simulink model "ActuatorLoop"  (R2019b)
settings: Solver=FixedStepDiscrete  StartTime=0.0  StopTime=10.0  FixedStep=0.001  RelTol=1e-3  EnableMultiTasking=on
model workspace (MAT data in the model file):
  Kd = Simulink.Parameter
  Kd.Value = 0.00272
  Kd.DataType = 'double'
  Kd.Dimensions = [1 1]
  Ki = Simulink.Parameter
  Ki.Value = 2.73
  Ki.DataType = 'double'
  Ki.Dimensions = [1 1]
  Kp = Simulink.Parameter
  Kp.Value = 0.339
  Kp.DataType = 'double'
  Kp.Dimensions = [1 1]
undefined symbols (not defined in the file or in its folder): DiscIntNeverNeededParam
libraries: simulink x2
Description:
  | This model implements a proportional, integral, derivative controller to close the loop on a hydraulic actuator.
settings Model: RequirementInfo="{}  %GIDa_c39459e1_b1c4_416b_a121_7cdfa8af617e"  DataDictionary=HeliSystemDD.sldd  ParameterArgumentNames=Kp,Kd,Ki  Creator=bpotter  LastModifiedBy=bpotter
settings DataIOCC: LimitDataPoints=on  SaveFormat=Array  SaveOutput=off  SignalLogging=off  DSMLogging=off  SaveTime=off
settings OptimizationCC: BlockReduction=off  DefaultParameterBehavior=Inlined  UseDivisionForNetSlopeComputation=on  InlineInvariantSignals=on  InitFltsAndDblsToZero=on  EfficientFloat2IntCast=on  EfficientMapNaN2IntZero=off  LifeSpan=inf  MaxStackSize=inf  EfficientTunableParamExpr=on
settings DebuggingCC: SignalInfNanChecking=error  SignalRangeChecking=error  ReadBeforeWriteMsg=EnableAllAsError  WriteAfterWriteMsg=EnableAllAsError  WriteAfterReadMsg=EnableAllAsError  AlgebraicLoopMsg=error  ArtificialAlgebraicLoopMsg=error  SaveWithDisabledLinksMsg=error  SaveWithParameterizedLinksMsg=error  BlockPriorityViolationMsg=error  SolverPrmCheckMsg=error  InheritedTsInSrcMsg=error  SingleTaskRateTransMsg=error  TasksWithSamePriorityMsg=error  SigSpecEnsureSampleTimeMsg=error  CheckMatrixSingularityMsg=error  IntegerOverflowMsg=error  ParameterUnderflowMsg=error  ParameterPrecisionLossMsg=error  ParameterTunabilityLossMsg=error  UnderSpecifiedDataTypeMsg=error  UnnecessaryDatatypeConvMsg=warning  VectorMatrixConversionMsg=error  SignalLabelMismatchMsg=error  UnconnectedInputMsg=error  UnconnectedOutputMsg=error  UnconnectedLineMsg=error  SFcnCompatibilityMsg=error  UniqueDataStoreMsg=error  BusObjectLabelMismatch=error  RootOutportRequireBusObject=error  AssertControl=DisableAll  AllowSymbolicDim=off  ModelReferenceIOMsg=error  ModelReferenceIOMismatchMessage=error  UnknownTsInhSupMsg=error  ModelReferenceDataLoggingMessage=error  StateNameClashWarn=warning  PregeneratedLibrarySubsystemCodeDiagnostic=none  StrictBusMsg=ErrorOnBusTreatedAsVector  NonBusSignalsTreatedAsBus=error  SFInvalidInputDataAccessInChartInitDiag=error  SFTransitionOutsideNaturalParentDiag=error  SFUnreachableExecutionPathDiag=error  SFUndirectedBroadcastEventsDiag=error  SFTransitionActionBeforeConditionDiag=error  SFExecutionAtInitializationDiag=none  IntegerSaturationMsg=error  ArithmeticOperatorsInVariantConditions=warning
settings HardwareCC: ProdBitPerPointer=32  ProdBitPerSizeT=32  ProdBitPerPtrDiffT=32  ProdWordSize=32  ProdHWDeviceType=Intel->x86-32 (Windows32)
settings ModelReferenceCC: PropagateSignalLabelsOutOfModel=off
settings SFSimCC: SimUseLocalCustomCode=off  CompileTimeRecursionLimit=0  EnableRuntimeRecursion=off  MATLABDynamicMemAlloc=off  CustomCodeUndefinedFunction=UseInterfaceOnly
settings RTWCC: SystemTargetFile=ert.tlc  TemplateMakefile=ert_default_tmf  GenerateReport=on  RTWUseLocalCustomCode=off  IncludeHyperlinkInReport=on  LaunchReport=on  PortableWordSizes=on  GenerateTraceInfo=on
settings CodeAppCC: ForceParamTrailComments=on  IgnoreCustomStorageClasses=off  MATLABFcnDesc=on  MangleLength=4  CustomSymbolStrModelFcn=$N  StateflowObjectComments=on  ReqsInCode=on
settings ERTTargetCC: TargetLangStandard=C99 (ISO)  UtilityFuncGeneration=Shared location  MultiwordLength=2048  GenerateSampleERTMain=on  IncludeMdlTerminateFcn=off  SuppressErrorStatus=on  SupportAbsoluteTime=off  SupportNonFinite=off  ParenthesesLevel=Maximum  CastingMode=Standards  GenerateSharedConstants=off  InlinedParameterPlacement=NonHierarchical  ERTCustomFileTemplate=example_file_process.tlc  ERTFilePackagingFormat=Compact  PreserveExpressionOrder=on  PreserveIfCondition=on  ConvertIfToSwitch=off  SuppressUnreachableDefaultCases=off  EnableSignedLeftShifts=off  EnableSignedRightShifts=off
settings ConfigComp: CovMetricSettings=dw  CovHtmlReporting=on  CovSaveCumulativeToWorkspaceVar=on  CovSaveSingleToWorkspaceVar=on  CovExternalEMLEnable=off  CovSFcnEnable=off  PSVerificationMode=BugFinder  PSResultDir=BugFinder_results_$ModelName$  PSAutoStubLUT=off

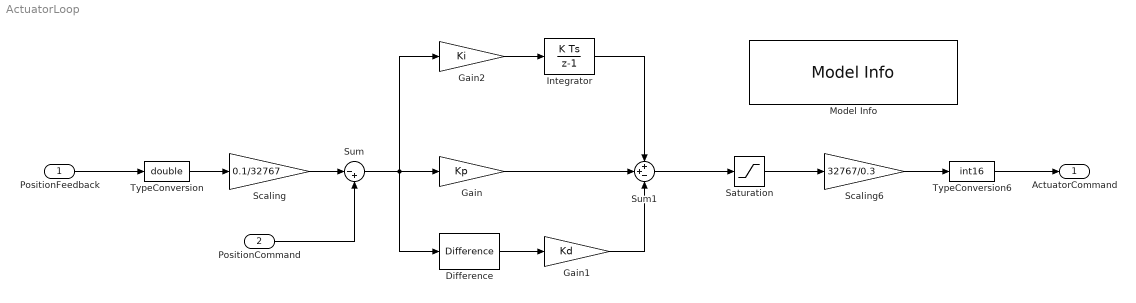
== system ActuatorLoop ==
  PositionFeedback : Inport  RequirementInfo={} %GIDa_7cfb5098_cfb3_4ea3_a772_b110fc5247af  OutMin=-32768  OutMax=32767  OutDataTypeStr=int16  PortDimensions=1  SampleTime=0.001
  PositionCommand : Inport  RequirementInfo={} %GIDa_6af42174_6d82_4ebc_8bab_c19e6798c116  Port=2  OutMin=-0.1  OutMax=0.1  OutDataTypeStr=double  PortDimensions=1  SampleTime=0.001
  Difference : simulink/Discrete/Difference  RequirementInfo={} %GIDa_90d6b033_9cb9_40c7_b35e_033491e477c9  ICPrevInput=0.0  OutMin=[]  OutMax=[]  OutDataType=fixdt(1, 16)  OutScaling=2^-10  DoSatur=off
  Gain : Gain  RequirementInfo={} %GIDa_81261c78_7d90_4c3c_8a54_887bf05a630d  Gain=Kp
  Gain1 : Gain  RequirementInfo={} %GIDa_5d7d8362_1967_4992_bb3b_38a72ebc61ca  Gain=Kd
  Gain2 : Gain  RequirementInfo={} %GIDa_1c3736c2_de3f_4491_b8cf_7dd8c6c6f71b  Gain=Ki
  Integrator : DiscreteIntegrator  RequirementInfo={} %GIDa_aa124dc7_6443_4cbb_bb02_1cdd6b45c090  SampleTime=-1  LimitOutput=on  UpperSaturationLimit=0.1  LowerSaturationLimit=-0.1  ICPrevOutput=DiscIntNeverNeededParam  ICPrevScaledInput=DiscIntNeverNeededParam
      settings: AttributesFormatString="%<LowerSaturationLimit> to  %<UpperSaturationLimit>"
  Model Info : simulink/Model-Wide Utilities/Model Info  Frame=on  DisplayStringWithTags=|  HorizontalTextAlignment=Center  LeftAlignmentValue=0.5
      | Model Name: %<ModelName>
      | Model Version: %<ModelVersion>
      | Last Modified: %<LastModificationDate>
      | 
      | Copyright 2016 The MathWorks, Inc.
  Saturation : Saturate  RequirementInfo={} %GIDa_8ac92945_a301_4fef_a0ea_5ecfd6c47c62  UpperLimit=0.3  LowerLimit=-0.3
      settings: AttributesFormatString=%<LowerLimit> to %<UpperLimit>
  Scaling : Gain  Gain=0.1/32767
  Scaling6 : Gain  Gain=32767/0.3  SaturateOnIntegerOverflow=on  OutDataTypeStr=Inherit: Same as input
  Sum : Sum  RequirementInfo={} %GIDa_d38775e8_f124_43a8_82cc_6598fe8ea0e4  Inputs=|-+
  Sum1 : Sum  RequirementInfo={} %GIDa_c0b02d8e_6114_4add_ae74_a5491d42d294  Inputs=++-
  TypeConversion : DataTypeConversion  OutDataTypeStr=double
  TypeConversion6 : DataTypeConversion  OutDataTypeStr=int16
  ActuatorCommand : Outport  RequirementInfo={} %GIDa_d1666590_09eb_4dbd_9180_483dbf5dbc22  VectorParamsAs1DForOutWhenUnconnected=off
  wires:
  PositionCommand/1 -> Sum/2
  Sum/1 -> Difference/1, Gain2/1, Gain/1
  Gain/1 -> Sum1/2
  Sum1/1 -> Saturation/1
  Integrator/1 -> Sum1/1
  Difference/1 -> Gain1/1
  Gain1/1 -> Sum1/3
  Gain2/1 -> Integrator/1
  PositionFeedback/1 -> TypeConversion/1
  TypeConversion/1 -> Scaling/1
  Scaling/1 -> Sum/1
  Scaling6/1 -> TypeConversion6/1
  Saturation/1 -> Scaling6/1
  TypeConversion6/1 -> ActuatorCommand/1
